simulink model "PerturbedCartesianOrbitPropagator"  (R2023a)
settings: Solver=ode4  StartTime=0.0  StopTime=10.0  FixedStep=6  RelTol=1e-3
settings Model: Creator=ndelurgio  LastModifiedBy=ndelurgio

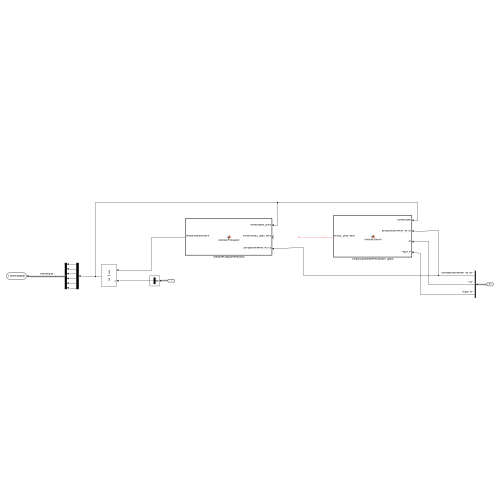
[thumbnail: Simulink's stored preview of the top-level diagram]
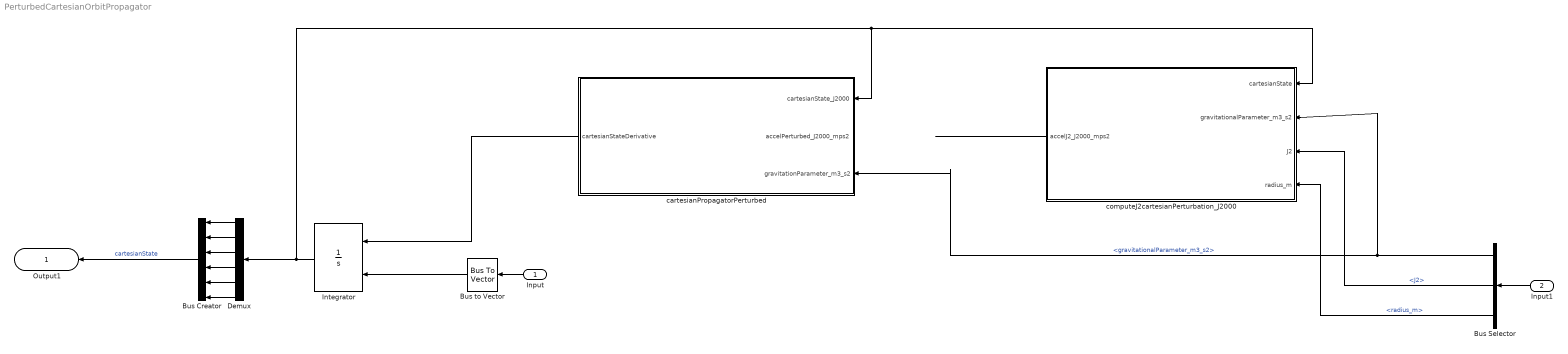
== system PerturbedCartesianOrbitPropagator ==
  Input : Inport  OutDataTypeStr=Bus: cartesianState
  Input1 : Inport  Port=2  OutDataTypeStr=Bus: earthProperties
  Bus Creator : BusCreator  Inputs=6  OutDataTypeStr=Bus: cartesianState  NonVirtualBus=on
      settings: InheritFromInputs=off
  Bus Selector : BusSelector  OutputSignals=gravitationalParameter_m3_s2,J2,radius_m
  Bus to Vector : BusToVector
  Demux : Demux  Outputs=6
  Integrator : Integrator  InitialConditionSource=external
  cartesianPropagatorPerturbed : MATLAB Function  TreatAsAtomicUnit=on
  computeJ2cartesianPerturbation_J2000 : MATLAB Function  TreatAsAtomicUnit=on
  Output1 : Outport  OutDataTypeStr=Bus: cartesianState
  wires:
  Input/1 -> Bus to Vector/1
  Bus to Vector/1 -> Integrator/2
  cartesianPropagatorPerturbed/1(cartesianStateDerivative) -> Integrator/1
  Integrator/1 -> Demux/1, computeJ2cartesianPerturbation_J2000/1(cartesianState), cartesianPropagatorPerturbed/1(cartesianState_J2000)
  computeJ2cartesianPerturbation_J2000/1(accelJ2_J2000_mps2) -> ?
  Input1/1 -> Bus Selector/1
  Bus Selector/1 -> cartesianPropagatorPerturbed/3(gravitationParameter_m3_s2), computeJ2cartesianPerturbation_J2000/2(gravitationalParameter_m3_s2)  "<gravitationalParameter_m3_s2>"
  Bus Selector/2 -> computeJ2cartesianPerturbation_J2000/3(J2)  "<J2>"
  Bus Selector/3 -> computeJ2cartesianPerturbation_J2000/4(radius_m)  "<radius_m>"
  Demux/2 -> Bus Creator/2
  Bus Creator/1 -> Output1/1  "cartesianState"
  Demux/3 -> Bus Creator/3
  Demux/1 -> Bus Creator/1
  Demux/6 -> Bus Creator/6
  Demux/5 -> Bus Creator/5
  Demux/4 -> Bus Creator/4

== matlab function PerturbedCartesianOrbitPropagator/cartesianPropagatorPerturbed ==
  data: cartesianState_J2000 input; cartesianStateDerivative output; accelPerturbed_J2000_mps2 input; gravitationParameter_m3_s2 input
function cartesianStateDerivative = cartesianPropagator(cartesianState_J2000,accelPerturbed_J2000_mps2,gravitationParameter_m3_s2)

cartesianStateDerivative = cartesianPropagatorPerturbed(cartesianState_J2000,accelPerturbed_J2000_mps2,gravitationParameter_m3_s2);

end

== matlab function PerturbedCartesianOrbitPropagator/computeJ2cartesianPerturbation_J2000 ==
  data: cartesianState input; accelJ2_J2000_mps2 output; gravitationalParameter_m3_s2 input; J2 input; radius_m input
function accelJ2_J2000_mps2 = computeJ2accel(cartesianState,gravitationalParameter_m3_s2,J2,radius_m)

accelJ2_J2000_mps2 = computeJ2cartesianPerturbation_J2000(cartesianState,gravitationalParameter_m3_s2,J2,radius_m);

end
